simulink model "test"  (Simulink 7.9)
settings: Solver=ode45  StartTime=0.0  StopTime=10.0  RelTol=1e-3
settings Model: Creator=hamid  LastModifiedBy=hamid

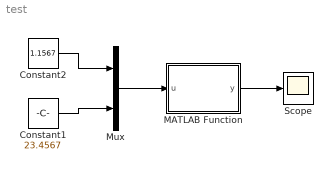
== system test ==
  Constant1 : Constant  Value=23.4567
  Constant2 : Constant  Value=1.1567
  MATLAB Function : MATLAB Function  TreatAsAtomicUnit=on
  Mux : Mux  Inputs=2
  Scope : Scope
  wires:
  Constant2/1 -> Mux/1
  Constant1/1 -> Mux/2
  Mux/1 -> MATLAB Function/1(u)
  MATLAB Function/1(y) -> Scope/1

== matlab function MATLAB Function ==
  data: u input double; y output double
function y = fcn(u)
 X=1:0.1:14';
Y=-5:0.1:35';
y = interp1(X,Y,u);
